simulink model "ExampleSimpleVehicleTyre"  (Simulink 9.2)
settings: Solver=FixedStepDiscrete  StartTime=0.0  StopTime=Inf  FixedStep=0.001  RelTol=1e-3  EnableMultiTasking=on
libraries: rFproPhysicsLib x14
settings Model: Creator=enewton  LastModifiedBy=SeanKavanagh  ParamWorkspaceSource=ReferencedWorkspace  TunableVars=LOCAL_PORT_RECV,REMOTE_PORT_RECV,gCGHeight,gFrontTrack,gFrontWheelRadius,gLeftWheelBase,gRearTrack,gRearWheelRadius,gRightWheelBase  TunableVarsStorageClass=Auto,Auto,Auto,Auto,Auto,Auto,Auto,Auto,Auto  TunableVarsTypeQualifier=,,,,,,,,
settings DataIOCC: SaveOutput=off  SignalLogging=off  DSMLogging=off  SaveTime=off
settings OptimizationCC: DefaultParameterBehavior=Inlined  ExpressionDepthLimit=2147483647
settings DebuggingCC: SolverPrmCheckMsg=warning  InheritedTsInSrcMsg=none
settings RTWCC: TargetLang=C++

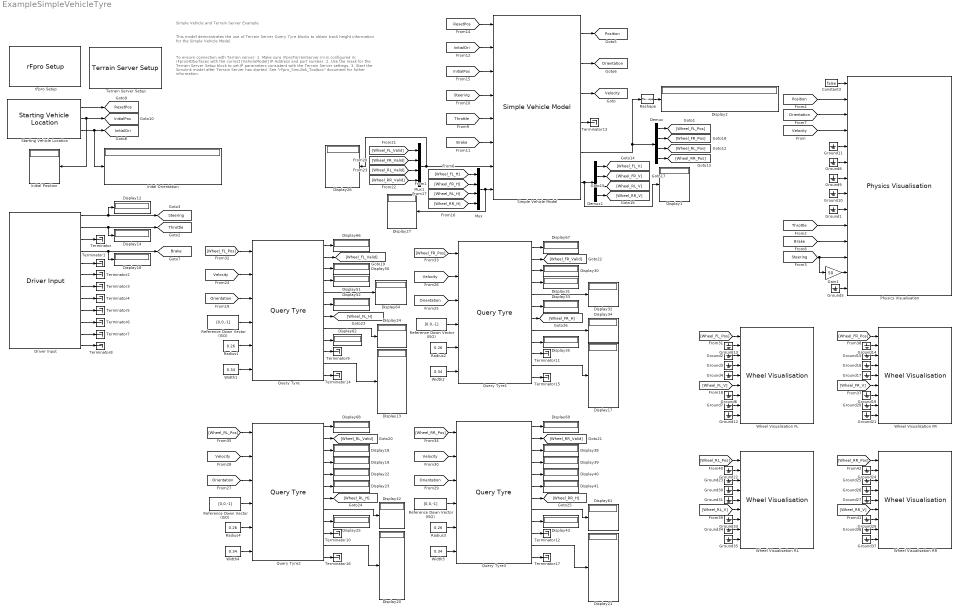
== system ExampleSimpleVehicleTyre ==
  note: To ensure connection with Terrain server:
      |
      | 1. Make sure rFproTerrainServer.ini is configured in: rFpro\HDSurfaces with the correct
      |     [VehicleModel] IP Address and port number.
      |
      | 2. Use the mask for the Terrain Server Setup block to set IP parameters consistent with
      |     the Terrain Server settings.
      |
      | 3. Start the Simulink model after Terrain Server has started.
      |
      | See "rFpro_Simulink_Toolbox" document for futher information.
  note: Simple Vehicle and Terrain Server Example
  note: This model demonstrates the use of Terrain Server Query Tyre blocks to obtain track height information
      | for the Simple Vehicle Model.
  Constant3 : Constant  Value=false
  Demux : Demux
  Demux1 : Demux
  Display{1..2,12..14,16..27,30..35,38..43,50..52,61..62,64,66..69} (39 alike) : Display
  Driver Input : rFproPhysicsLib/Driver Input
  Gain1 : Gain  Gain=50
  Ground{1..17,19..27,29..31,33..37} (34 alike) : Ground
  Inital Orientation : Display
  Initial Position : Display
  Mux : Mux
  Mux1 : Mux
  Physics Visualisation : rFproPhysicsLib/Physics Visualisation  PAR_SKIP_INTERNAL_PHYSICS=off  PAR_ACCEL_VALID=off  PAR_ROT_ACCEL_VALID=off  PAR_GEAR_VALID=off  PAR_RPM_VALID=off  PAR_INPUTS_VALID=on  PAR_STEER_TORQUE_VALID=on  PAR_HEADLIGHTS_ON_VALID=off  PAR_WHEEL_POS_VALID=on  PAR_WHEEL_ORI_VALID=off  PAR_TYRE_PARAMS_VALID=off  PAR_WHEEL_ROTATION_VALID=on  PAR_WHEEL_BRAKE_TEMP_VALID=off  PAR_WHEEL_TREAD_TEMP_VALID=off  PAR_WHEEL_AIR_TEMP_VALID=off  period=-1  offset=0  useReverseByteOrder=on  rFpro__platform=Remote Model - Default
  Query Tyre : rFproPhysicsLib/Terrain Server Blocks/Query Tyre  wheel=FL  iso_mode=on  sampletime=-1  phase_delay=0  roundtrip_frames=2  numUserDataElements=0  useReverseByteOrder=off  rFpro__TS_platform=Remote Model - Default  msgSize=0
  Query Tyre1 : rFproPhysicsLib/Terrain Server Blocks/Query Tyre  wheel=FR  iso_mode=on  sampletime=-1  phase_delay=0  roundtrip_frames=2  numUserDataElements=0  useReverseByteOrder=off  rFpro__TS_platform=Remote Model - Default  msgSize=0
  Query Tyre2 : rFproPhysicsLib/Terrain Server Blocks/Query Tyre  wheel=RL  iso_mode=on  sampletime=-1  phase_delay=0  roundtrip_frames=2  numUserDataElements=0  useReverseByteOrder=off  rFpro__TS_platform=Remote Model - Default  msgSize=0
  Query Tyre3 : rFproPhysicsLib/Terrain Server Blocks/Query Tyre  wheel=RR  iso_mode=on  sampletime=-1  phase_delay=0  roundtrip_frames=2  numUserDataElements=0  useReverseByteOrder=off  rFpro__TS_platform=Remote Model - Default  msgSize=0
  Radius{1..4} (4 alike) : Constant  Value=0.26  OutDataTypeStr=double
  Reference Down Vector (ISO) : Constant  Value=[0,0,-1]
  "Reference Down Vector (ISO) " : Constant  Value=[0,0,-1]
  "Reference Down Vector (ISO)  " : Constant  Value=[0,0,-1]
  "Reference Down Vector (ISO)   " : Constant  Value=[0,0,-1]
  Reshape : Reshape  OutputDimensionality=Customize  OutputDimensions=[3,4]
  Simple Vehicle Model : rFproPhysicsLib/Internal Utility/Simple Vehicle Model  TIMESTEP=-1  gCGHeight=0.52  gLeftWheelBase=2.626  gRightWheelBase=2.626  gFrontTrack=1.55  gRearTrack=1.525  gFrontWheelRadius=0.32  gRearWheelRadius=0.33  gWheelDeflection=0
  Starting Vehicle Location : rFproPhysicsLib/Starting Vehicle Location  cg_offset=CG_OFFSET_FROM_NOSE  numPackets=1  rFpro__platform=Remote Model - Default
  Terminator{,1..17} (18 alike) : Terminator
  Terrain Server Setup : rFproPhysicsLib/Terrain Server Blocks/Terrain Server Setup  Priority=0  track_name=''  tyre_config=[]  points_config=[]  iso=on  triggerOnHeartbeat=off  heartbeat_latency=750  rFpro__platform=Remote Model - Default  ts_address='127.0.0.1'  ts_port=11006  sendSampleTime=-1  sl_address='127.0.0.1'  sl_port=11002  receiveSampleTime=-1  maxUDPMsgs=3  useReverseByteOrder=off
  Wheel Visualisation FL : rFproPhysicsLib/Wheel Visualisation  wheelStr=FL
  Wheel Visualisation FR : rFproPhysicsLib/Wheel Visualisation  wheelStr=FR
  Wheel Visualisation RL : rFproPhysicsLib/Wheel Visualisation  wheelStr=RL
  Wheel Visualisation RR : rFproPhysicsLib/Wheel Visualisation  wheelStr=RR
  Width{1..4} (4 alike) : Constant  Value=0.34  OutDataTypeStr=double
  rFpro Setup : rFproPhysicsLib/rFpro Setup  platform=Remote Model - Default  stopOnSessionEnd=on  usePseudoRealtime=on  syncToRF=on  useReverseByteOrder=off  useRfTime=on  minIterations=4  maxIterations=1000  ipReceiveAddress='127.0.0.1'  ipReceivePort=11054  receiveSampleTime=-1  ipTransmitAddress='127.0.0.1'  ipTransmitPort=11052  transmitSampleTime=-1  pluginType=RUN_PHYSICS  sysTarget=xpctarget.tlc  templateMakeFile=xpc_default_tmf  makeCommand=make_rtw  buildDesc=xPC target
  tag scope: Brake=global, InitialOri=global, InitialPos=global, Orientation=global, Position=global, ResetPos=global, Steering=global, Throttle=global, Velocity=global
  wires:
  Starting Vehicle Location/3 -> [InitialOri], Inital Orientation/1
  Starting Vehicle Location/2 -> Initial Position/1, [InitialPos]
  Constant3/1 -> Physics Visualisation/1
  [Orientation] -> Physics Visualisation/3
  [Velocity] -> Physics Visualisation/4
  [Throttle] -> Physics Visualisation/10
  [Steering] -> Physics Visualisation/12, Gain1/1
  [Brake] -> Physics Visualisation/11
  Driver Input/1 -> [Steering], Display12/1
  Driver Input/2 -> [Throttle], Display14/1
  Driver Input/4 -> [Brake], Display16/1
  [Position] -> Physics Visualisation/2
  Driver Input/3 -> Terminator/1
  Driver Input/5 -> Terminator1/1
  Driver Input/6 -> Terminator2/1
  Driver Input/7 -> Terminator3/1
  Driver Input/8 -> Terminator4/1
  Driver Input/9 -> Terminator5/1
  Driver Input/10 -> Terminator6/1
  Driver Input/11 -> Terminator7/1
  Driver Input/12 -> Terminator8/1
  Ground8/1 -> Physics Visualisation/6
  Ground9/1 -> Physics Visualisation/7
  Ground10/1 -> Physics Visualisation/8
  Ground11/1 -> Physics Visualisation/5
  Starting Vehicle Location/1 -> [ResetPos]
  Gain1/1 -> Physics Visualisation/13
  Ground2/1 -> Wheel Visualisation FL/3
  Ground3/1 -> Wheel Visualisation FL/4
  Ground4/1 -> Wheel Visualisation FL/5
  [Wheel_FL_V] -> Wheel Visualisation FL/6
  Ground6/1 -> Wheel Visualisation FL/7
  Ground7/1 -> Wheel Visualisation FL/8
  Ground12/1 -> Wheel Visualisation FL/9
  Ground13/1 -> Wheel Visualisation FL/2
  Ground14/1 -> Wheel Visualisation FR/2
  Ground15/1 -> Wheel Visualisation FR/3
  Ground16/1 -> Wheel Visualisation FR/4
  Ground17/1 -> Wheel Visualisation FR/5
  Ground19/1 -> Wheel Visualisation FR/7
  Ground20/1 -> Wheel Visualisation FR/8
  Ground21/1 -> Wheel Visualisation FR/9
  Ground22/1 -> Wheel Visualisation RL/2
  Ground23/1 -> Wheel Visualisation RL/3
  Ground30/1 -> Wheel Visualisation RL/4
  Ground31/1 -> Wheel Visualisation RL/5
  Ground33/1 -> Wheel Visualisation RL/7
  Ground34/1 -> Wheel Visualisation RL/8
  Ground35/1 -> Wheel Visualisation RL/9
  Ground24/1 -> Wheel Visualisation RR/2
  Ground25/1 -> Wheel Visualisation RR/3
  Ground26/1 -> Wheel Visualisation RR/4
  Ground27/1 -> Wheel Visualisation RR/5
  Ground29/1 -> Wheel Visualisation RR/7
  Ground36/1 -> Wheel Visualisation RR/8
  Ground37/1 -> Wheel Visualisation RR/9
  Reference Down Vector (ISO)/1 -> Query Tyre/4
  Query Tyre/2 -> [Wheel_FL_Valid]
  Query Tyre/4 -> Display51/1
  Query Tyre/6 -> Display52/1
  Query Tyre/3 -> Display50/1
  [Orientation] -> Query Tyre/3
  [Velocity] -> Query Tyre1/2
  [Orientation] -> Query Tyre1/3
  "Reference Down Vector (ISO)  "/1 -> Query Tyre1/4
  [Velocity] -> Query Tyre2/2
  [Orientation] -> Query Tyre2/3
  "Reference Down Vector (ISO) "/1 -> Query Tyre2/4
  [Velocity] -> Query Tyre3/2
  [Orientation] -> Query Tyre3/3
  "Reference Down Vector (ISO)   "/1 -> Query Tyre3/4
  Query Tyre2/2 -> [Wheel_RL_Valid]
  Query Tyre2/3 -> Display18/1
  Query Tyre2/4 -> Display19/1
  Query Tyre2/5 -> Display22/1
  Query Tyre2/6 -> Display23/1
  Query Tyre2/9 -> Display25/1
  Query Tyre2/10 -> Terminator10/1
  Query Tyre1/2 -> [Wheel_FR_Valid]
  Query Tyre1/3 -> Display30/1
  Query Tyre1/4 -> Display31/1
  Query Tyre1/5 -> Display32/1
  Query Tyre1/6 -> Display33/1
  Query Tyre1/9 -> Display35/1
  Query Tyre1/10 -> Terminator11/1
  Query Tyre3/2 -> [Wheel_RR_Valid]
  Query Tyre3/3 -> Display38/1
  Query Tyre3/4 -> Display39/1
  Query Tyre3/5 -> Display40/1
  Query Tyre3/6 -> Display41/1
  Query Tyre3/9 -> Display43/1
  Query Tyre3/10 -> Terminator12/1
  [Velocity] -> Query Tyre/2
  Query Tyre/9 -> Display62/1
  Query Tyre/10 -> Terminator9/1
  Query Tyre/5 -> Display64/1
  Query Tyre/8 -> Display24/1
  Query Tyre1/8 -> Display34/1
  Query Tyre2/8 -> Display42/1
  Query Tyre3/8 -> Display61/1
  Query Tyre/1 -> Display66/1
  Query Tyre1/1 -> Display67/1
  Query Tyre2/1 -> Display68/1
  Query Tyre3/1 -> Display69/1
  Simple Vehicle Model/1 -> [Position]
  Simple Vehicle Model/2 -> [Orientation]
  Simple Vehicle Model/3 -> [Velocity]
  [Throttle] -> Simple Vehicle Model/5
  [InitialPos] -> Simple Vehicle Model/3
  [Steering] -> Simple Vehicle Model/4
  [ResetPos] -> Simple Vehicle Model/1
  [Brake] -> Simple Vehicle Model/6
  [InitialOri] -> Simple Vehicle Model/2
  Simple Vehicle Model/5 -> Demux/1, Reshape/1
  Demux/1 -> [Wheel_FL_Pos]
  Demux/2 -> [Wheel_FR_Pos]
  Demux/3 -> [Wheel_RL_Pos]
  Demux/4 -> [Wheel_RR_Pos]
  Demux1/1 -> [Wheel_FL_V]
  Demux1/2 -> [Wheel_FR_V]
  Demux1/3 -> [Wheel_RL_V]
  Demux1/4 -> [Wheel_RR_V]
  Simple Vehicle Model/6 -> Display1/1, Demux1/1
  [Wheel_RL_Valid] -> Mux1/3
  [Wheel_RR_Valid] -> Mux1/4
  [Wheel_FL_Valid] -> Mux1/1
  [Wheel_FR_Valid] -> Mux1/2
  [Wheel_FR_H] -> Mux/2
  [Wheel_FL_H] -> Mux/1
  [Wheel_RR_H] -> Mux/4
  [Wheel_RL_H] -> Mux/3
  Mux1/1 -> Display26/1, Simple Vehicle Model/7
  Mux/1 -> Display27/1, Simple Vehicle Model/8
  [Wheel_FL_Pos] -> Wheel Visualisation FL/1
  [Wheel_FR_Pos] -> Wheel Visualisation FR/1
  [Wheel_FR_V] -> Wheel Visualisation FR/6
  [Wheel_RL_Pos] -> Wheel Visualisation RL/1
  [Wheel_RL_V] -> Wheel Visualisation RL/6
  [Wheel_RR_Pos] -> Wheel Visualisation RR/1
  [Wheel_RR_V] -> Wheel Visualisation RR/6
  [Wheel_FL_Pos] -> Query Tyre/1
  [Wheel_RL_Pos] -> Query Tyre2/1
  [Wheel_FR_Pos] -> Query Tyre1/1
  [Wheel_RR_Pos] -> Query Tyre3/1
  Query Tyre/7 -> [Wheel_FL_H]
  Query Tyre2/7 -> [Wheel_RL_H]
  Query Tyre1/7 -> [Wheel_FR_H]
  Query Tyre3/7 -> [Wheel_RR_H]
  Query Tyre/11 -> Display13/1
  Query Tyre1/11 -> Display17/1
  Query Tyre2/11 -> Display20/1
  Query Tyre3/11 -> Display21/1
  Ground5/1 -> Physics Visualisation/14
  Reshape/1 -> Display2/1
  Radius1/1 -> Query Tyre/5
  Width1/1 -> Query Tyre/6
  Radius4/1 -> Query Tyre2/5
  Width4/1 -> Query Tyre2/6
  Width3/1 -> Query Tyre3/6
  Radius3/1 -> Query Tyre3/5
  Radius2/1 -> Query Tyre1/5
  Width2/1 -> Query Tyre1/6
  Ground1/1 -> Physics Visualisation/9
  Simple Vehicle Model/4 -> Terminator13/1
  Query Tyre/12 -> Terminator14/1
  Query Tyre1/12 -> Terminator15/1
  Query Tyre2/12 -> Terminator16/1
  Query Tyre3/12 -> Terminator17/1
